simulink model "discrete_nonlinear"  (R2017b)
settings: Solver=VariableStepAuto  StartTime=0.0  StopTime=100  RelTol=1e-3
values from neighbouring files (symbols this model uses):
  a1 = 0.44    [workspace.mat]    (also in workspace2.mat)
  a2 = 0.51    [workspace.mat]    (also in workspace2.mat)
  a3 = 0.48    [workspace.mat]    (also in workspace2.mat)
  a4 = -0.65    [workspace.mat]    (also in workspace2.mat)
  K = 2.5    [workspace.mat]    (also in workspace2.mat)
  T1 = 5    [workspace.mat]    (also in workspace2.mat)
  T2 = 10    [workspace.mat]    (also in workspace2.mat)
  Tp = 1    [workspace.mat]    (also in workspace2.mat)
settings Model: Creator=gulin  LastModifiedBy=gulin

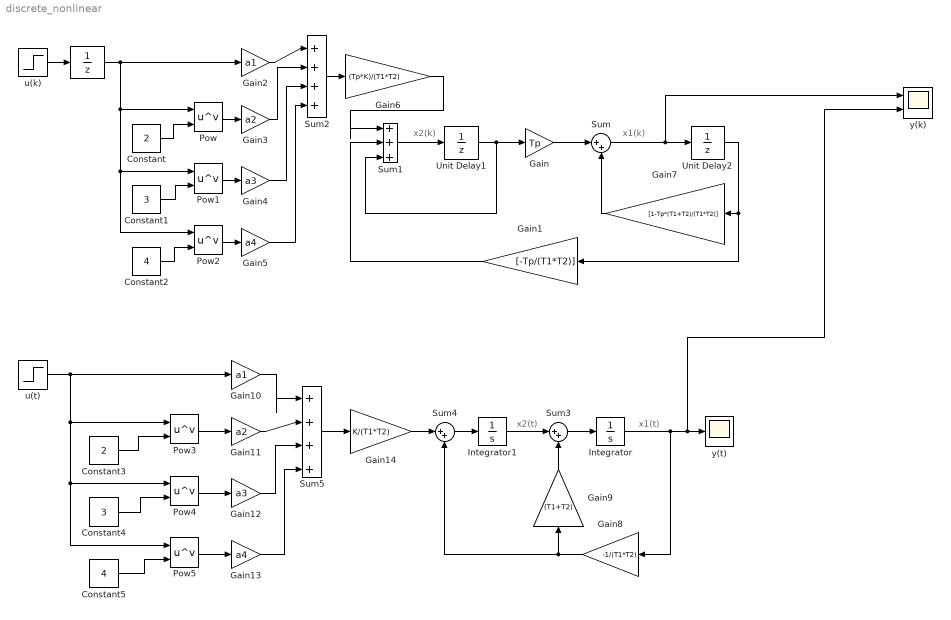
== system discrete_nonlinear ==
  note: x1(k)
  note: x2(k)
  note: x2(t)
  note: x1(t)
  " " : UnitDelay  SampleTime=-1
  Constant : Constant  Value=2
  Constant1 : Constant  Value=3
  Constant2 : Constant  Value=4
  Constant3 : Constant  Value=2
  Constant4 : Constant  Value=3
  Constant5 : Constant  Value=4
  Gain : Gain  Gain=Tp
  Gain1 : Gain  Gain=[-Tp/(T1*T2)]
  Gain10 : Gain  Gain=a1
  Gain11 : Gain  Gain=a2
  Gain12 : Gain  Gain=a3
  Gain13 : Gain  Gain=a4
  Gain14 : Gain  Gain=K/(T1*T2)
  Gain2 : Gain  Gain=a1
  Gain3 : Gain  Gain=a2
  Gain4 : Gain  Gain=a3
  Gain5 : Gain  Gain=a4
  Gain6 : Gain  Gain=(Tp*K)/(T1*T2)
  Gain7 : Gain  Gain=[1-Tp*(T1+T2)/(T1*T2)]
  Gain8 : Gain  Gain=-1/(T1*T2)
  Gain9 : Gain  Gain=(T1+T2)
  Integrator : Integrator
  Integrator1 : Integrator
  Pow{,1..5} (6 alike) : Math  Operator=pow  RndMeth=Zero  SaturateOnIntegerOverflow=on
  Sum : Sum  Inputs=|++
  Sum1 : Sum  Inputs=|+++
  Sum2 : Sum  Inputs=|++++
  Sum3 : Sum  Inputs=|++
  Sum4 : Sum  Inputs=|++
  Sum5 : Sum  Inputs=|++++
  Unit Delay1 : UnitDelay  SampleTime=-1
  Unit Delay2 : UnitDelay  SampleTime=-1
  u(k) : Step  SampleTime=0
  "u(t) " : Step  SampleTime=0
  y(k) : Scope  NumInputPorts=2
  "y(t) " : Scope
  wires:
  Gain4/1 -> Sum2/3
  Gain3/1 -> Sum2/2
  Pow1/1 -> Gain4/1
  Constant2/1 -> Pow2/2
  Pow2/1 -> Gain5/1
  Constant/1 -> Pow/2
  u(k)/1 -> " "/1
  Gain2/1 -> Sum2/1
  Gain5/1 -> Sum2/4
  Constant1/1 -> Pow1/2
  Sum2/1 -> Gain6/1
  Pow/1 -> Gain3/1
  " "/1 -> Gain2/1, Pow2/1, Pow1/1, Pow/1
  Sum1/1 -> Unit Delay1/1
  Unit Delay1/1 -> Sum1/3, Gain/1
  Gain/1 -> Sum/1
  Sum/1 -> Unit Delay2/1, y(k)/1
  Gain6/1 -> Sum1/1
  Gain1/1 -> Sum1/2
  Pow5/1 -> Gain13/1
  Pow4/1 -> Gain12/1
  Gain11/1 -> Sum5/2
  Sum5/1 -> Gain14/1
  Sum4/1 -> Integrator1/1
  Gain14/1 -> Sum4/1
  Pow3/1 -> Gain11/1
  Constant4/1 -> Pow4/2
  Gain8/1 -> Gain9/1, Sum4/2
  "u(t) "/1 -> Pow5/1, Pow4/1, Pow3/1, Gain10/1
  Gain13/1 -> Sum5/4
  Constant3/1 -> Pow3/2
  Gain10/1 -> Sum5/1
  Integrator/1 -> y(k)/2, "y(t) "/1, Gain8/1
  Constant5/1 -> Pow5/2
  Integrator1/1 -> Sum3/1
  Gain9/1 -> Sum3/2
  Sum3/1 -> Integrator/1
  Gain12/1 -> Sum5/3
  Unit Delay2/1 -> Gain1/1, Gain7/1
  Gain7/1 -> Sum/2
